simulink model "blink_challenge_sim"  (R2015a)
settings: Solver=FixedStepDiscrete  StartTime=0.0  StopTime=60.0  RelTol=1e-3
libraries: arduino_io_lib x9, simulink x5
settings Model: Creator=gcampa  LastModifiedBy=Osman
settings DataIOCC: SignalLoggingSaveFormat=ModelDataLogs
settings OptimizationCC: ExpressionDepthLimit=2147483647
settings DebuggingCC: UnderspecifiedInitializationDetection=Classic  MergeDetectMultiDrivingBlocksExec=none  SolverPrmCheckMsg=warning  FcnCallInpInsideContextMsg=UseLocalSettings  StateNameClashWarn=warning
settings HardwareCC: ProdBitPerInt=16  ProdBitPerPointer=16  ProdIntDivRoundTo=Zero  ProdEndianess=LittleEndian  ProdWordSize=8  ProdHWDeviceType=Atmel->AVR  TargetLongLongMode=on  TargetIntDivRoundTo=Zero  TargetEndianess=LittleEndian  TargetHWDeviceType=MATLAB Host  ProdEqTarget=off
settings RTWCC: SystemTargetFile=rsim.tlc  TemplateMakefile=rsim_default_tmf  Description=Rapid Simulation Target
settings RSimTargetCC: ERTMultiwordTypeDef=System defined  ERTMultiwordLength=256

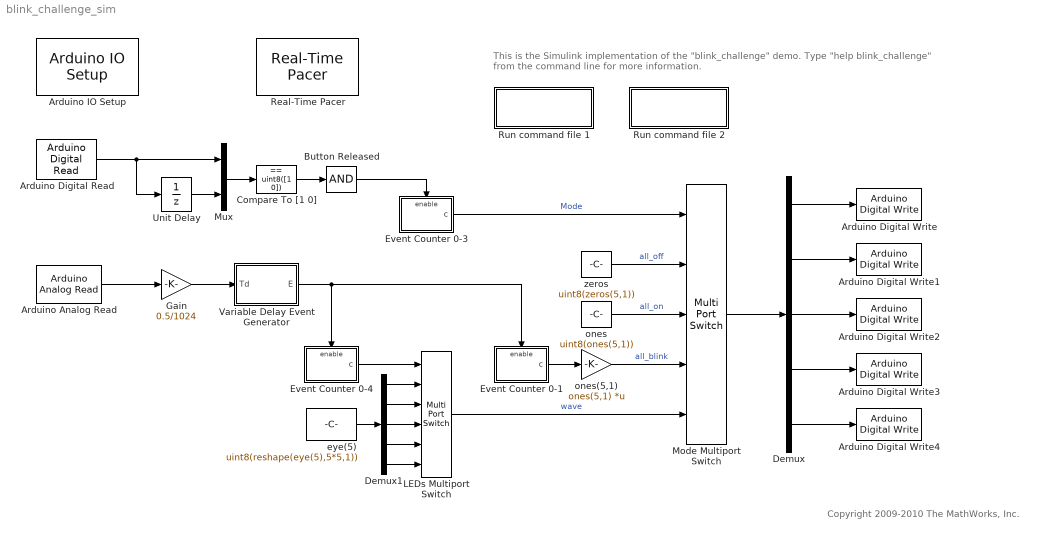
== system blink_challenge_sim ==
  note: This is the Simulink implementation of the "blink_challenge" demo.
      |   Type "help blink_challenge" from the command line for more information.
  note: Copyright 2009-2010 The MathWorks, Inc.
  Arduino Analog Read : arduino_io_lib/Arduino Analog Read  arduinoVar=Temporary arduino variable: Arduino1  arduinoPin=2  T=0.1
  Arduino Digital Read : arduino_io_lib/Arduino Digital Read  arduinoVar=Temporary arduino variable: Arduino1  arduinoPin=2  T=0.1
  Arduino Digital Write : arduino_io_lib/Arduino Digital Write  arduinoVar=Temporary arduino variable: Arduino1  arduinoPin=9  T=-1
  Arduino Digital Write1 : arduino_io_lib/Arduino Digital Write  arduinoVar=Temporary arduino variable: Arduino1  arduinoPin=10  T=-1
  Arduino Digital Write2 : arduino_io_lib/Arduino Digital Write  arduinoVar=Temporary arduino variable: Arduino1  arduinoPin=11  T=-1
  Arduino Digital Write3 : arduino_io_lib/Arduino Digital Write  arduinoVar=Temporary arduino variable: Arduino1  arduinoPin=12  T=-1
  Arduino Digital Write4 : arduino_io_lib/Arduino Digital Write  arduinoVar=Temporary arduino variable: Arduino1  arduinoPin=13  T=-1
  Arduino IO Setup : arduino_io_lib/Arduino IO Setup  Priority=3  arduinoVar=Temporary arduino variable: Arduino1  workspaceVarName=a  comPort=COM9
  Button Released : Logic  Inputs=1  AllPortsSameDT=off  OutDataTypeStr=boolean
  Compare To [1 0] : simulink/Logic and Bit Operations/Compare To Constant  relop===  const=uint8([1 0])  OutDataTypeStr=uint8
  Demux : Demux  Outputs=ones(5,1)
  Demux1 : Demux  Outputs=5*ones(5,1)
  Event Counter 0-1 : Subsystem  mask(Event Counter){L=1}
      mask prompts: L "Upper Limit"
      mask help: Every time the block is enabled and evaluated, the counter increments the output variable, which wraps to zero after reaching the limit.
      mask Help: Every time the block is enabled and evaluated, the counter increments the output variable, which wraps to zero after reaching the limit.
  Event Counter 0-3 : Subsystem  mask(Event Counter){L=3}
      mask prompts: L "Upper Limit"
      mask help: Every time the block is enabled and evaluated, the counter increments the output variable, which wraps to zero after reaching the limit.
      mask Help: Every time the block is enabled and evaluated, the counter increments the output variable, which wraps to zero after reaching the limit.
  Event Counter 0-4 : Subsystem  mask(Event Counter){L=4}
      mask prompts: L "Upper Limit"
      mask help: Every time the block is enabled and evaluated, the counter increments the output variable, which wraps to zero after reaching the limit.
      mask Help: Every time the block is enabled and evaluated, the counter increments the output variable, which wraps to zero after reaching the limit.
  Gain : Gain  Gain=0.5/1024
  LEDs Multiport Switch : MultiPortSwitch  DataPortOrder=Zero-based contiguous  Inputs=5  zeroidx=on
  Mode Multiport Switch : MultiPortSwitch  DataPortOrder=Zero-based contiguous  Inputs=4  zeroidx=on
  Mux : Mux  Inputs=[1 1]
  Real-Time Pacer : arduino_io_lib/Real-Time Pacer  simTimePerRealTime=1
  Run command file 1 : Subsystem
      settings: OpenFcn=blink_challenge_sf
      mask Display: disp('Stateflow \nImplementation')
  Run command file 2 : Subsystem
      settings: OpenFcn=edit('blink_challenge.m');
      mask Display: disp('MATLAB \nImplementation')
  Unit Delay : UnitDelay  SampleTime=-1
  Variable Delay Event Generator : Subsystem  mask(Variable Delay Event Generator){T=0.1}
      mask prompts: T "Sampling Time (T)"
      mask help:
      | The input (Td) is a constant scalar expressing the desired delay between events.
      | Every Td seconds the output goes to 1 and then it goes back to zero after T seconds.
      mask init:
      | if T<=0, error('The sampling time of the "Variable Delay Event Generator" block must be greater than 0'); end
      mask Help:
      | The input (Td) is a constant scalar expressing the desired delay between events.
      | Every Td seconds the output goes to 1 and then it goes back to zero after T seconds.
  eye(5) : Constant  Value=uint8(reshape(eye(5),5*5,1))
  ones : Constant  Value=uint8(ones(5,1))
  ones(5,1) : Gain  Gain=ones(5,1)  Multiplication=Matrix(K*u)  OutDataTypeStr=uint8
  zeros : Constant  Value=uint8(zeros(5,1))
  wires:
  Demux/1 -> Arduino Digital Write/1
  Demux/2 -> Arduino Digital Write1/1
  Demux/3 -> Arduino Digital Write2/1
  Demux/4 -> Arduino Digital Write3/1
  Demux/5 -> Arduino Digital Write4/1
  Arduino Analog Read/1 -> Gain/1
  Arduino Digital Read/1 -> Unit Delay/1, Mux/1
  Mode Multiport Switch/1 -> Demux/1
  Unit Delay/1 -> Mux/2
  Mux/1 -> Compare To [1 0]/1
  Compare To [1 0]/1 -> Button Released/1
  Button Released/1 -> Event Counter 0-3/Enable
  Event Counter 0-1/1(c) -> ones(5,1)/1
  ones(5,1)/1 -> Mode Multiport Switch/4  "all_blink"
  zeros/1 -> Mode Multiport Switch/2  "all_off"
  ones/1 -> Mode Multiport Switch/3  "all_on"
  LEDs Multiport Switch/1 -> Mode Multiport Switch/5  "wave"
  Event Counter 0-3/1(c) -> Mode Multiport Switch/1  "Mode"
  Demux1/1 -> LEDs Multiport Switch/2
  Demux1/2 -> LEDs Multiport Switch/3
  Demux1/3 -> LEDs Multiport Switch/4
  Demux1/4 -> LEDs Multiport Switch/5
  Demux1/5 -> LEDs Multiport Switch/6
  eye(5)/1 -> Demux1/1
  Gain/1 -> Variable Delay Event Generator/1(Td)
  Variable Delay Event Generator/1(E) -> Event Counter 0-1/Enable, Event Counter 0-4/Enable
  Event Counter 0-4/1(c) -> LEDs Multiport Switch/1

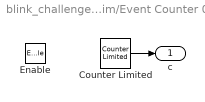
== system blink_challenge_sim/Event Counter 0-1 ==
  Enable : EnablePort
  Counter Limited : simulink/Sources/Counter Limited  SystemSampleTime=-1  uplimit=L  tsamp=-1
  c : Outport  InitialOutput=0
  wires:
  Counter Limited/1 -> c/1

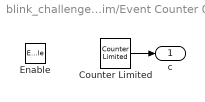
== system blink_challenge_sim/Event Counter 0-3 ==
  Enable : EnablePort
  Counter Limited : simulink/Sources/Counter Limited  SystemSampleTime=-1  uplimit=L  tsamp=-1
  c : Outport  InitialOutput=0
  wires:
  Counter Limited/1 -> c/1

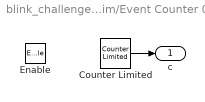
== system blink_challenge_sim/Event Counter 0-4 ==
  Enable : EnablePort
  Counter Limited : simulink/Sources/Counter Limited  SystemSampleTime=-1  uplimit=L  tsamp=-1
  c : Outport  InitialOutput=0
  wires:
  Counter Limited/1 -> c/1

== system blink_challenge_sim/Run command file 1 ==

== system blink_challenge_sim/Run command file 2 ==

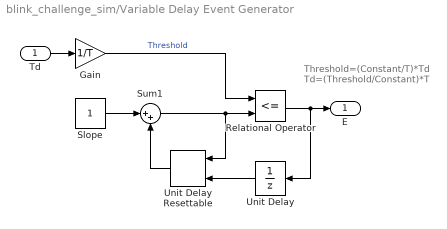
== system blink_challenge_sim/Variable Delay Event Generator ==
  note: Threshold=(Constant/T)*Td
      | Td=(Threshold/Constant)*T
  Td : Inport
  Gain : Gain  Gain=1/T
  Relational Operator : RelationalOperator  Operator=<=  OutDataTypeStr=boolean
  Slope : Constant  SampleTime=T
  Sum1 : Sum  Inputs=|++
  Unit Delay : UnitDelay  InitialCondition=uint8(0)  SampleTime=-1
  Unit Delay Resettable : simulink/Additional Math & Discrete/Additional Discrete/Unit Delay Resettable  SystemSampleTime=-1  vinit=0.0  tsamp=-1
  E : Outport
  wires:
  Td/1 -> Gain/1
  Gain/1 -> Relational Operator/1  "Threshold"
  Unit Delay/1 -> Unit Delay Resettable/2
  Relational Operator/1 -> E/1, Unit Delay/1
  Slope/1 -> Sum1/1
  Sum1/1 -> Unit Delay Resettable/1, Relational Operator/2
  Unit Delay Resettable/1 -> Sum1/2
